simulink model "s_cd_hmc_v3_dsim"  (R2016b)
(part 24 of 59)

  Gateway Out36/1 -> To Workspace52/1
  Gateway Out40/1 -> To Workspace53/1
  Gateway Out43/1 -> To Workspace55/1
  Gateway Out44/1 -> To Workspace56/1
  Gateway Out45/1 -> To Workspace57/1
  Gateway Out50/1 -> To Workspace58/1
  cd_hmc_clear_tp1/1(sim_out) -> To Workspace61/1
  Constant26/1 -> Relational2/2
  Register3/1 -> cd_hmc_clear_tp1/1(out_reg)
  Relational2/1 -> Register3/3, Register3/1
  cd_hmc_clear_tp2/1(sim_out) -> To Workspace62/1
  Register6/1 -> cd_hmc_clear_tp2/1(out_reg)
  Relational3/1 -> Register6/3, Register6/1
  Constant31/1 -> Relational3/2
  addr1/1 -> write_addr_gen_lnk3/1(addr_in), write_addr_gen_lnk2/1(addr_in), Gateway Out156/1, Relational2/1, Relational3/1, Relational/1
  cd_hmc_clear_tp3/1(sim_out) -> To Workspace63/1
  Register7/1 -> cd_hmc_clear_tp3/1(out_reg)
  Relational4/1 -> Register7/1, Register7/3
  Constant27/1 -> Relational4/2
  [hmc_clear_wraddr_pol1] -> Relational4/1
  edge_detect22/1 -> Register8/2, Register7/2, Register6/2, Register3/2, addr_stall1/1, Register/2, Register2/2, reord_clear/1, addr1/1, Gateway Out116/1
  cd_hmc_clear_tp4/1(sim_out) -> To Workspace64/1
  Register8/1 -> cd_hmc_clear_tp4/1(out_reg)
  Relational6/1 -> Register8/3, Register8/1
  Constant32/1 -> Relational6/2
  [hmc_clear_wraddr_pol0] -> Relational6/1
  [hmc_clear_done] -> Inverter4/1
  Inverter4/1 -> Logical7/3
  hmc/16 -> pipeline277/1(d)
  hmc/15 -> pipeline280/1(d)
  hmc/14 -> pipeline283/1(d)
  hmc/13 -> pipeline284/1(d)
  pipeline284/1(q) -> [rx_crc_err_lnk2]
  pipeline283/1(q) -> [rx_crc_err_lnk3]
  pipeline280/1(q) -> [errstat_lnk2]
  pipeline277/1(q) -> [errstat_lnk3]
  rx_crc_err_lnk2/1(sim_out) -> To Workspace65/1
  [rx_crc_err_lnk2] -> rx_crc_err_lnk2/1(out_reg)
  rx_crc_err_lnk3/1(sim_out) -> To Workspace66/1
  [rx_crc_err_lnk3] -> rx_crc_err_lnk3/1(out_reg)
  [errstat_lnk3] -> errstat_lnk3/1(out_reg)
  [errstat_lnk2] -> errstat_lnk2/1(out_reg)
  errstat_lnk2/1(sim_out) -> To Workspace78/1
  errstat_lnk3/1(sim_out) -> To Workspace79/1
  [reord_clear_wea] -> Gateway Out120/1, Mux10/2
  Gateway Out60/1 -> To Workspace87/1
  Gateway Out61/1 -> To Workspace88/1
  Logical18/1 -> Reorder_cntrl/1(rst)
  [local_rst] -> Logical18/1
  edge_detect/1 -> Logical18/2
  [hmc_dvalid] -> Gateway Out121/1, Mux10/3
  [hmc_dout] -> Gateway Out52/1, Mux9/3
  [hmc_tag_out] -> Gateway Out48/1, Mux8/3
  hmc_wr_err_p1/1(sim_out) -> To Workspace1/1
  Counter1/1 -> pipeline4/1(d)
  pipeline4/1(q) -> hmc_wr_err_p1/1(out_reg)
  pipeline6/1(q) -> Counter1/1
  [sync_mon_rst] -> edge_detect2/1
  [hmc_wr_rdy_pol1] -> Inverter1/1
  Inverter1/1 -> Logical2/1
  pipeline7/1(q) -> Counter1/2
  Logical2/1 -> pipeline7/1(d)
  hmc_rd_err_p1/1(sim_out) -> To Workspace2/1
  Counter2/1 -> pipeline8/1(d)
  pipeline8/1(q) -> hmc_rd_err_p1/1(out_reg)
  pipeline13/1(q) -> Counter2/1
  [sync_mon_rst] -> edge_detect1/1
  [hmc_rd_rdy_pol1] -> Inverter3/1
  Inverter3/1 -> Logical3/1
  pipeline14/1(q) -> Counter2/2
  Logical3/1 -> pipeline14/1(d)
  edge_detect1/1 -> pipeline13/1(d)
  edge_detect2/1 -> pipeline6/1(d)
  [hmc_win_p1] -> Logical2/2
  [hmc_rin_p1] -> Logical3/2
  hmc_wr_rd_rdy_clash_p1/1(sim_out) -> To Workspace5/1
  Counter3/1 -> pipeline15/1(d)
  pipeline15/1(q) -> hmc_wr_rd_rdy_clash_p1/1(out_reg)
  pipeline18/1(q) -> Counter3/1
  pipeline26/1(q) -> Counter3/2
  [sync_mon_rst] -> edge_detect3/1
  [hmc_rd_rdy_pol1] -> Logical4/2
  [hmc_wr_rdy_pol1] -> Logical4/1
  Logical4/1 -> pipeline26/1(d)
  edge_detect3/1 -> pipeline18/1(d)
  [reord_data_in] -> Slice1/1
  Delay3/1 -> bus_expand/1(bus_in)
  Delay5/1 -> edge_detect4/1, reord_din/11(in_dv), reord_din/13(we)
  [reord_wea] -> Delay5/1
  Delay12/1 -> edge_detect5/1, reorda/9(we)
  [reord_wea] -> Delay12/1
  Slice1/1 -> Delay3/1
  edge_detect4/1 -> reord_din/14(trig), reord_din/12(in_sync)
  [reord_addr] -> Delay7/1
  [reord_bram_en_pol0] -> Delay15/1
  Delay7/1 -> reorda/1(in_addra)
  Delay18/1 -> reorda/2(in_addrb)
  [reord_bram_rd_add_pol0] -> Delay18/1
  [reord_wea] -> Delay14/1
  Delay14/1 -> reorda/3(in_ena)
  Delay15/1 -> reorda/4(in_enb)
  [Pol0_reord_rdy_phase1] -> Delay19/1
  [Pol0_reord_rdy_phase2] -> Delay20/1
  [Pol1_reord_rdy_phase1] -> Delay22/1
  [Pol1_reord_rdy_phase2] -> Delay26/1
  Delay19/1 -> reorda/5(in_p0_ph1_rdy)
  Delay20/1 -> reorda/6(in_p0_ph2_rdy)
  Delay22/1 -> reorda/7(in_p1_ph1_rdy)
  Delay26/1 -> reorda/8(in_p1_ph2_rdy)
  edge_detect5/1 -> reorda/10(trig)
  [hmc_reord_data] -> Slice2/1
  Delay27/1 -> bus_expand1/1(bus_in)
  Delay29/1 -> reord_dout/9(in_dv), reord_dout/11(we)
  [hmc_reord_dvalid] -> Delay29/1
  Slice2/1 -> Delay27/1
  [hmc_reord_sync] -> Delay30/1
  Delay30/1 -> reord_dout/10(in_sync), reord_dout/12(trig)
  [reord_addr] -> Delay40/1
  Delay40/1 -> reord_din/9(in_addra)
  Delay41/1 -> reord_din/10(in_ena)
  [reord_wea] -> Delay41/1
  Delay34/1 -> edge_detect6/1, reordb/7(we)
  [reord_bram_en_pol0] -> Delay34/1
  [reord_bram_en_pol0] -> Delay38/1
  Delay38/1 -> reordb/2(in_enb)
  [Pol0_reord_rdy_phase1] -> Delay42/1
  [Pol0_reord_rdy_phase2] -> Delay43/1
  [Pol1_reord_rdy_phase1] -> Delay44/1
  [Pol1_reord_rdy_phase2] -> Delay45/1
  Delay42/1 -> reordb/3(in_p0_ph1_rdy)
  Delay43/1 -> reordb/4(in_p0_ph2_rdy)
  Delay44/1 -> reordb/5(in_p1_ph1_rdy)
  Delay45/1 -> reordb/6(in_p1_ph2_rdy)
  edge_detect6/1 -> reordb/8(trig)
  [reord_bram_rd_add_pol0] -> Delay35/1
  Delay35/1 -> reordb/1(in_addrb)
  bus_expand/1(msb_out8) -> reord_din/1(in_d0)
  bus_expand/2(out7) -> reord_din/2(in_d1)
  bus_expand/3(out6) -> reord_din/3(in_d2)
  bus_expand/4(out5) -> reord_din/4(in_d3)
  bus_expand/5(out4) -> reord_din/5(in_d4)
  bus_expand/6(out3) -> reord_din/6(in_d5)
  bus_expand/7(out2) -> reord_din/7(in_d6)
  bus_expand/8(lsb_out1) -> reord_din/8(in_d7)
  bus_expand1/1(msb_out8) -> reord_dout/1(in_d0)
  bus_expand1/2(out7) -> reord_dout/2(in_d1)
  bus_expand1/3(out6) -> reord_dout/3(in_d2)
  bus_expand1/4(out5) -> reord_dout/4(in_d3)
  bus_expand1/5(out4) -> reord_dout/5(in_d4)
  bus_expand1/6(out3) -> reord_dout/6(in_d5)
  bus_expand1/7(out2) -> reord_dout/7(in_d6)
  bus_expand1/8(lsb_out1) -> reord_dout/8(in_d7)
  Gateway Out8/1 -> To Workspace9/1
  Gateway Out11/1 -> To Workspace11/1
  Gateway Out13/1 -> To Workspace12/1
  bus_expand2/3(out6) -> Gateway Out13/1
  bus_expand2/2(out7) -> Gateway Out11/1
  bus_expand2/1(msb_out8) -> Gateway Out8/1
  Gateway Out14/1 -> To Workspace13/1
  bus_expand2/4(out5) -> Gateway Out14/1
  Gateway Out18/1 -> To Workspace15/1
  bus_expand2/5(out4) -> Gateway Out18/1
  Gateway Out22/1 -> To Workspace16/1
  bus_expand2/6(out3) -> Gateway Out22/1
  Gateway Out24/1 -> To Workspace17/1
  bus_expand2/7(out2) -> Gateway Out24/1
  Gateway Out25/1 -> To Workspace18/1
  bus_expand2/8(lsb_out1) -> Gateway Out25/1
  Gateway Out32/1 -> To Workspace10/1
  Gateway Out26/1 -> To Workspace22/1
  bus_expand3/3(out6) -> Gateway Out26/1
  bus_expand3/2(out7) -> Gateway Out9/1
  bus_expand3/1(msb_out8) -> Gateway Out32/1
  Gateway Out27/1 -> To Workspace23/1
  bus_expand3/4(out5) -> Gateway Out27/1
  Gateway Out28/1 -> To Workspace24/1
  bus_expand3/5(out4) -> Gateway Out28/1
  Gateway Out29/1 -> To Workspace25/1
  bus_expand3/6(out3) -> Gateway Out29/1
  Gateway Out30/1 -> To Workspace26/1
  bus_expand3/7(out2) -> Gateway Out30/1
  Gateway Out31/1 -> To Workspace27/1
  bus_expand3/8(lsb_out1) -> Gateway Out31/1
  Slice4/1 -> bus_expand3/1(bus_in)
  Gateway Out46/1 -> To Workspace19/1
  Gateway Out47/1 -> To Workspace28/1
  Gateway Out33/1 -> To Workspace29/1
  bus_expand4/3(out6) -> Gateway Out33/1
  bus_expand4/2(out7) -> Gateway Out47/1
  bus_expand4/1(msb_out8) -> Gateway Out46/1
  Gateway Out35/1 -> To Workspace31/1
  bus_expand4/4(out5) -> Gateway Out35/1
  Gateway Out37/1 -> To Workspace32/1
  bus_expand4/5(out4) -> Gateway Out37/1
  Gateway Out38/1 -> To Workspace33/1
  bus_expand4/6(out3) -> Gateway Out38/1
  Gateway Out39/1 -> To Workspace34/1
  bus_expand4/7(out2) -> Gateway Out39/1
  Gateway Out42/1 -> To Workspace35/1
  bus_expand4/8(lsb_out1) -> Gateway Out42/1
  Slice3/1 -> bus_expand4/1(bus_in)
  Gateway Out9/1 -> To Workspace21/1
  Gateway Out48/1 -> To Workspace36/1
  Gateway Out49/1 -> To Workspace39/1
  [reord_data_in] -> Gateway Out51/1, Slice4/1, Slice3/1
  Gateway Out51/1 -> To Workspace40/1
  Gateway Out52/1 -> To Workspace41/1
  Gateway Out53/1 -> To Workspace42/1
  Gateway Out54/1 -> To Workspace44/1
  Gateway Out55/1 -> To Workspace45/1
  Gateway Out65/1 -> To Workspace50/1
  Gateway Out56/1 -> To Workspace70/1
  bus_expand5/3(out6) -> Gateway Out56/1
  bus_expand5/2(out7) -> Gateway Out75/1
  bus_expand5/1(msb_out8) -> Gateway Out65/1
  Gateway Out58/1 -> To Workspace71/1
  bus_expand5/4(out5) -> Gateway Out58/1
  Gateway Out59/1 -> To Workspace72/1
  bus_expand5/5(out4) -> Gateway Out59/1
  Gateway Out62/1 -> To Workspace73/1
  bus_expand5/6(out3) -> Gateway Out62/1
  Gateway Out63/1 -> To Workspace74/1
  bus_expand5/7(out2) -> Gateway Out63/1
  Gateway Out64/1 -> To Workspace77/1
  bus_expand5/8(lsb_out1) -> Gateway Out64/1
  Slice6/1 -> bus_expand5/1(bus_in)
  Gateway Out72/1 -> To Workspace47/1
  Gateway Out73/1 -> To Workspace46/1
  Gateway Out66/1 -> To Workspace48/1
  bus_expand6/3(out6) -> Gateway Out66/1
  bus_expand6/2(out7) -> Gateway Out73/1
  bus_expand6/1(msb_out8) -> Gateway Out72/1
  Gateway Out67/1 -> To Workspace49/1
  bus_expand6/4(out5) -> Gateway Out67/1
  Gateway Out68/1 -> To Workspace59/1
  bus_expand6/5(out4) -> Gateway Out68/1
  Gateway Out69/1 -> To Workspace60/1
  bus_expand6/6(out3) -> Gateway Out69/1
  Gateway Out70/1 -> To Workspace67/1
  bus_expand6/7(out2) -> Gateway Out70/1
  Gateway Out71/1 -> To Workspace68/1
  bus_expand6/8(lsb_out1) -> Gateway Out71/1
  Slice5/1 -> bus_expand6/1(bus_in)
  Gateway Out75/1 -> To Workspace69/1
  [hmc_reord_data] -> Slice5/1, Slice6/1, Gateway Out74/1
  Gateway Out74/1 -> To Workspace81/1
  Gateway Out76/1 -> To Workspace82/1
  Gateway Out77/1 -> To Workspace83/1
  Gateway Out88/1 -> To Workspace98/1
  bus_expand7/3(out6) -> Gateway Out78/1
  bus_expand7/2(out7) -> Gateway Out100/1
  bus_expand7/1(msb_out8) -> Gateway Out88/1
  bus_expand7/4(out5) -> Gateway Out79/1
  bus_expand7/5(out4) -> Gateway Out80/1
  bus_expand7/6(out3) -> Gateway Out81/1
  bus_expand7/7(out2) -> Gateway Out86/1
  bus_expand7/8(lsb_out1) -> Gateway Out87/1
  Gateway Out98/1 -> To Workspace85/1
  Gateway Out99/1 -> To Workspace86/1
  Gateway Out89/1 -> To Workspace89/1
  bus_expand8/3(out6) -> Gateway Out89/1
  bus_expand8/2(out7) -> Gateway Out99/1
  bus_expand8/1(msb_out8) -> Gateway Out98/1
  Gateway Out90/1 -> To Workspace90/1
  bus_expand8/4(out5) -> Gateway Out90/1
  Gateway Out92/1 -> To Workspace94/1
  bus_expand8/5(out4) -> Gateway Out92/1
  Gateway Out94/1 -> To Workspace95/1
  bus_expand8/6(out3) -> Gateway Out94/1
  Gateway Out95/1 -> To Workspace96/1
  bus_expand8/7(out2) -> Gateway Out95/1
  Gateway Out97/1 -> To Workspace97/1
  bus_expand8/8(lsb_out1) -> Gateway Out97/1
  Gateway Out78/1 -> To Workspace99/1
  Gateway Out79/1 -> To Workspace100/1
  Gateway Out80/1 -> To Workspace101/1
  Gateway Out81/1 -> To Workspace102/1
  Gateway Out86/1 -> To Workspace103/1
  Gateway Out87/1 -> To Workspace104/1
  Gateway Out100/1 -> To Workspace105/1
  Slice7/1 -> bus_expand8/1(bus_in)
  Slice8/1 -> bus_expand7/1(bus_in)
  Gateway Out119/1 -> To Workspace115/1
  bus_expand9/3(out6) -> Gateway Out102/1
  bus_expand9/2(out7) -> Gateway Out101/1
  bus_expand9/1(msb_out8) -> Gateway Out119/1
  bus_expand9/4(out5) -> Gateway Out103/1
  bus_expand9/5(out4) -> Gateway Out104/1
  bus_expand9/6(out3) -> Gateway Out105/1
  bus_expand9/7(out2) -> Gateway Out115/1
  bus_expand9/8(lsb_out1) -> Gateway Out118/1
  Gateway Out102/1 -> To Workspace107/1
  Gateway Out103/1 -> To Workspace109/1
  Gateway Out104/1 -> To Workspace112/1
  Gateway Out105/1 -> To Workspace114/1
  Gateway Out115/1 -> To Workspace116/1
  Gateway Out118/1 -> To Workspace117/1
  Gateway Out101/1 -> To Workspace106/1
  Slice9/1 -> bus_expand9/1(bus_in)
  Delay9/1 -> [hmc_reord_dvalid], Gateway Out180/1
  Gateway Out120/1 -> To Workspace84/1
  Gateway Out121/1 -> To Workspace118/1
  Reorder_cntrl/2(bram_rd_en) -> Delay9/1, [reord_bram_en_pol0], Gateway Out7/1, HMC_reord_bram/7
  [hmc_reord_data] -> Slice10/1
  Delay39/1 -> bus_expand10/1(bus_in)
  Delay46/1 -> reord_dout1/11(we), reord_dout1/9(in_dv)
  [hmc_reord_dvalid] -> Delay46/1
  Slice10/1 -> Delay39/1
  [hmc_reord_sync] -> Delay47/1
  Delay47/1 -> reord_dout1/12(trig), reord_dout1/10(in_sync)
  bus_expand10/1(msb_out8) -> reord_dout1/1(in_d0)
  bus_expand10/2(out7) -> reord_dout1/2(in_d1)
  bus_expand10/3(out6) -> reord_dout1/3(in_d2)
  bus_expand10/4(out5) -> reord_dout1/4(in_d3)
  bus_expand10/5(out4) -> reord_dout1/5(in_d4)
  bus_expand10/6(out3) -> reord_dout1/6(in_d5)
  bus_expand10/7(out2) -> reord_dout1/7(in_d6)
  bus_expand10/8(lsb_out1) -> reord_dout1/8(in_d7)
  [reord_data_in] -> Slice11/1
  Delay48/1 -> bus_expand11/1(bus_in)
  Delay51/1 -> reord_din1/13(we), reord_din1/11(in_dv), edge_detect7/1
  [reord_wea] -> Delay51/1
  Slice11/1 -> Delay48/1
  edge_detect7/1 -> reord_din1/12(in_sync), reord_din1/14(trig)
  [reord_addr] -> Delay49/1
  Delay49/1 -> reord_din1/9(in_addra)
  Delay50/1 -> reord_din1/10(in_ena)
  [reord_wea] -> Delay50/1
  bus_expand11/1(msb_out8) -> reord_din1/1(in_d0)
  bus_expand11/2(out7) -> reord_din1/2(in_d1)
  bus_expand11/3(out6) -> reord_din1/3(in_d2)
  bus_expand11/4(out5) -> reord_din1/4(in_d3)
  bus_expand11/5(out4) -> reord_din1/5(in_d4)
  bus_expand11/6(out3) -> reord_din1/6(in_d5)
  bus_expand11/7(out2) -> reord_din1/7(in_d6)
  bus_expand11/8(lsb_out1) -> reord_din1/8(in_d7)
  reord_sync_out_upper/1(sim_out) -> To Workspace119/1
  Counter4/1 -> pipeline29/1(d)
  pipeline29/1(q) -> reord_sync_out_upper/1(out_reg)
  pipeline27/1(q) -> Counter4/1
  pipeline28/1(q) -> Counter4/2
  edge_detect8/1 -> pipeline27/1(d)
  reord_sync_out_lower/1(sim_out) -> To Workspace120/1
  Counter5/1 -> pipeline32/1(d)
  pipeline32/1(q) -> reord_sync_out_lower/1(out_reg)
  pipeline30/1(q) -> Counter5/1
  pipeline31/1(q) -> Counter5/2
  edge_detect10/1 -> pipeline30/1(d)
  [sync_mon_rst] -> edge_detect10/1, edge_detect8/1
  pipeline1/1(q) -> Delay36/1
  Delay4/1 -> AddSub/1, Delay1/1
  second/1 -> Delay25/1
  Delay13/1 -> second/1
  d/1 -> pipeline206/1(d)  "d_in"
  [dout] -> Delay6/1
  addr/1 -> Gateway Out12/1, Delay4/1  "addr"
  addr_stall/1 -> edge_detect9/1(in)  "stall"
  pipeline159/1(q) -> Gateway Out3/1, [radd]
  pipeline162/1(q) -> Gateway Out91/1, [din]
  Gateway Out19/1 -> To Workspace4/1
  pipeline199/1(q) -> [rin], Gateway Out4/1
  Delay28/1 -> Delay31/1
  Gateway Out1/1 -> To Workspace6/1
  Gateway Out2/1 -> To Workspace7/1
  Gateway Out3/1 -> To Workspace8/1
  Gateway Out4/1 -> To Workspace20/1
  pipeline9/1(q) -> Logical27/1
  Logical31/1 -> pipeline50/1(d)
  pipeline2/1(q) -> [hmc_delay]
  pipeline206/1(q) -> [dout]
  pipeline12/1(q) -> Delay23/1
  Delay36/1 -> Delay33/1
  AddSub/1 -> Delay32/1  "rd_add_HR"
  pipeline209/1(q) -> [hmc_sync], Gateway Out19/1
  Delay33/1 -> pipeline209/1(d)
  Delay32/1 -> pipeline159/1(d)
  Delay31/1 -> pipeline232/1(d), pipeline199/1(d)
  Delay25/1 -> pipeline162/1(d)
  Logical27/1 -> addr_stall/2
  [sync_in] -> pipeline1/1(d)
  en/1 -> Gateway Out140/1, [en_in]  "en_in"
  Delay70/1 -> pipeline233/1(d)
  AddSub2/1 -> Gateway Out181/1, AddSub/2
  Constant/1 -> AddSub2/2
  [delay_in] -> AddSub2/1
  pipeline232/1(q) -> Gateway Out2/1, [win]
  delay/1 -> Register13/1, Gateway Out176/1  "delay"
  Register13/1 -> Gateway Out166/1, [delay_in], pipeline2/1(d)
  Gateway Out91/1 -> To Workspace125/1
  pipeline233/1(q) -> Gateway Out1/1, [wadd]
  Delay1/1 -> Delay70/1
  Delay6/1 -> Delay13/1
  sync/1 -> [sync_in]  "sync_in"
  Gateway Out140/1 -> To Workspace168/1
  Delay23/1 -> Delay10/1
  Gateway Out166/1 -> To Workspace193/1
  Gateway Out175/1 -> To Workspace201/1
  [ld_val] -> edge_detect30/1(in)
  Gateway Out176/1 -> To Workspace202/1
  edge_detect30/1(out) -> Register13/3, Gateway Out175/1
  [en_in] -> pipeline9/1(d), pipeline12/1(d)
  Gateway Out181/1 -> To Workspace208/1
  [hmc_post] -> Logical31/2
  [hmc_clear_done] -> Logical31/3
  [hmc_init] -> Logical31/1
  edge_detect9/1(out) -> Convert2/1
  Gateway Out10/1 -> To Workspace3/1
  Gateway Out12/1 -> To Workspace14/1
  pipeline50/1(q) -> Logical27/2
  [local_rst] -> Gateway Out57/1, addr_stall/1, addr/1
  Delay10/1 -> second/3
  [local_rst] -> second/2
  [local_rst] -> Register13/2
  Gateway Out57/1 -> To Workspace80/1
  [sys_rst] -> Logical10/1
  [sync_in] -> Logical10/2
  Logical10/1 -> [local_rst]
  Convert2/1 -> Delay28/1, Gateway Out10/1, addr/2
  [local_rst] -> Logical11/3
